simulink model "ELM_tictactoe_V2"  (R2021b)
settings: Solver=VariableStepAuto  StartTime=0.0  StopTime=inf  RelTol=1e-3
(part 1 of 136)
settings Model: Creator=benwa  LastModifiedBy=benwa
settings SolverCC: AutoInsertRateTranBlk=on

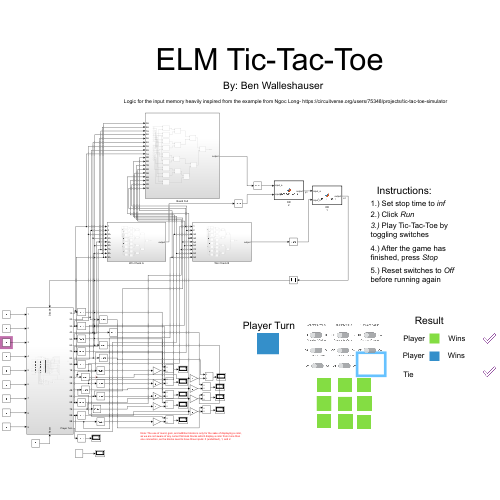
[thumbnail: Simulink's stored preview of the top-level diagram]
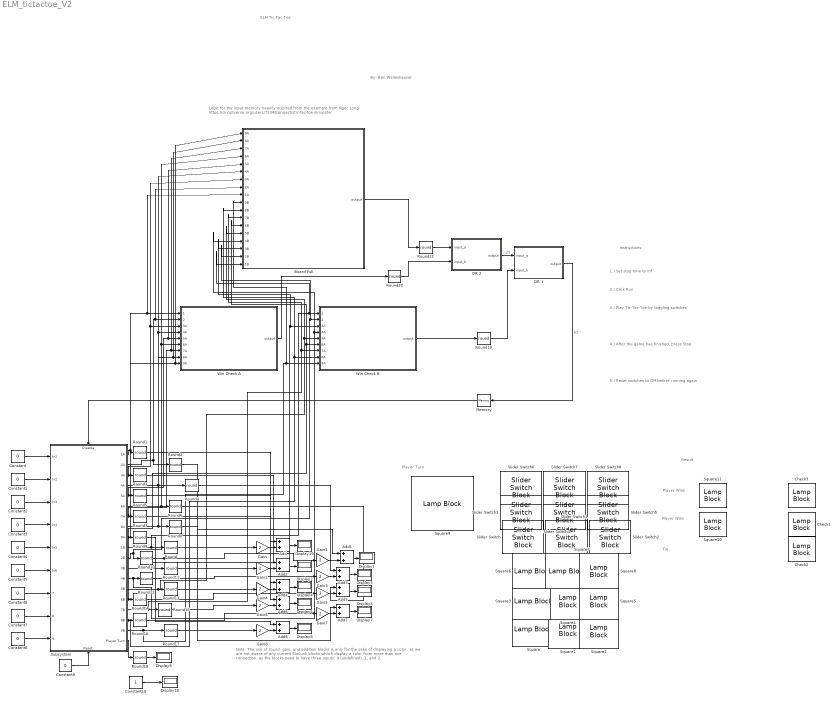
== system ELM_tictactoe_V2 ==
  note: Logic for the input memory heavily inspired from the example from Ngoc Long- https://circuitverse.org/users/75348/projects/tic-tac-toe-simulator
  note: By: Ben Walleshauser
  note: ELM Tic-Tac-Toe
  note: Note: The use of round, gain, and addition blocks is only for the sake of displaying a color, as we are not aware of any current Simlunk blocks whiich display a color from more than one connection, as the blocks need to have three inputs: 0 (undefined), 1, and 2.
  note: 1.) Set stop time to inf
  note: Instructions:
  note: Tie
  note: Player Wins
  note: Result
  note: Player Turn
  note: Player Wins
  note: 2.) Click Run
  note: 3.) Play Tic-Tac-Toe by toggling switches
  note: 4.) After the game has finished, press Stop
  note: 5.) Reset switches to Off before running again
  Add{,1..8} (9 alike) : Sum
  Board Full : Subsystem
  Check1 : LampBlock  LabelPosition=Hide  Icon=Check3
  Check2 : LampBlock  LabelPosition=Hide  Icon=Check3
  Check3 : LampBlock  LabelPosition=Hide  Icon=Check3
  Constant{,1..9} (10 alike) : Constant  Value=0
  Constant10 : Constant
  Display{1..10,19} (11 alike) : Display
  Gain{,1..8} (9 alike) : Gain  Gain=2
  Memory : Memory
  OR 1 : MATLAB Function  TreatAsAtomicUnit=on
  OR 2 : MATLAB Function  TreatAsAtomicUnit=on
  Round{,1..21} (22 alike) : Rounding  Operator=round
  Slider Switch{,1..8} (9 alike) : SliderSwitchBlock
      settings: Values={{'Off', 'On'}, [0 1]}
  Square{,1..11} (12 alike) : LampBlock  LabelPosition=Hide  Icon=Square
  Subsystem : Subsystem
      settings: PortSchema="{\"entries\":[{\"content\":{\"sides\":[{\"content\":{\"connectorIds\":[\"In1\",\"In2\",\"In3\",\"In4\",\"In5\",\"In6\",\"In7\",\"In8\",\"In9\"]},\"type\":\"ConnectorPlacement.EquallySpacedRectSide\",\"uuid\":\"24eea2ca-bc54-45b4-8ca7-8e6d0582f2d8\"},{\"content\":{\"connectorIds\":[\"Out1\",\"Out2\",\"Out3\",\"Out4\",\"Out5\",\"Out6\",\"Out7\",\"Out8\",\"Out9\",\"Out10\",\"Out11\",\"Out12\",\"Out13\",\"Out14\",\"Out15\",\"Out16\",\"Out17\",\"Out18\",\"Out19\"],\"side\":\"RIGHT\"},\"type\":\"ConnectorPlacement.EquallySpacedRectSide\",\"uuid\":\"dcdda681-f03f-4783-934e-bb305b550037\"},{\"content\":{\"connectorIds\":[\"In10\"],\"side\":\"TOP\"},\"type\":\"ConnectorPlacement.EquallySpacedRectSide\",\"uuid\":\"fbafddca-e088-423f-ae92-9e95b73c1056\"},{\"content\":{\"connectorIds\":[\"In11\"],\"side\":\"BOTTOM\"},\"type\":\"ConnectorPlacement.EquallySpacedRectSide\",\"uuid\":\"e1bf0a8c-befc-41e7-9839-13c2c519b1eb\"}]},\"type\":\"ConnectorPlacement.EquallySpacedConnector\",\"uuid\":\"afff88fe-c887-456a-b96a-e3a40750e04a\"}],\"packageUris\":[\"http://schema.mathworks.com/mf0/Connector/R2020b\"],\"version\":\"1.0\"}"
  Win Check A : Subsystem
  Win Check B : Subsystem
  wires:
  Constant/1 -> Subsystem/1(In1)
  Constant1/1 -> Subsystem/2(In2)
  Constant2/1 -> Subsystem/3(In3)
  Constant3/1 -> Subsystem/4(In4)
  Constant4/1 -> Subsystem/5(In5)
  Constant5/1 -> Subsystem/6(In6)
  Constant6/1 -> Subsystem/7(7)
  Constant7/1 -> Subsystem/8(8)
  Constant8/1 -> Subsystem/9(9)
  Constant9/1 -> Subsystem/11(Reset)
  Subsystem/1(1A) -> Round1/1, Board Full/9(1A), Win Check A/1(1)
  Subsystem/2(2A) -> Round2/1, Board Full/8(2A), Win Check A/2(2)
  Subsystem/3(3A) -> Board Full/7(3A), Win Check A/3(3A), Round3/1
  Subsystem/4(4A) -> Board Full/6(4A), Win Check A/4(4A), Round4/1
  Subsystem/5(5A) -> Board Full/5(5A), Win Check A/5(5A), Round5/1
  Subsystem/6(6A) -> Board Full/4(6A), Win Check A/6(6A), Round6/1
  Subsystem/7(7A) -> Board Full/3(7A), Win Check A/7(7A), Round7/1
  Subsystem/8(8A) -> Board Full/2(8A), Win Check A/8(8A), Round8/1
  Subsystem/9(9A) -> Round9/1, Board Full/1(9A), Win Check A/9(9A)
  Subsystem/10(1B) -> Win Check B/1(1), Board Full/18(1B), Round/1
  Subsystem/11(2B) -> Round10/1, Win Check B/2(2), Board Full/17(2B)
  Subsystem/12(3B) -> Win Check B/3(3A), Board Full/16(3B), Round11/1
  Subsystem/13(4B) -> Win Check B/4(4A), Board Full/15(4B), Round12/1
  Subsystem/14(5B) -> Win Check B/5(5A), Board Full/14(5B), Round13/1
  Subsystem/15(6B) -> Win Check B/6(6A), Board Full/13(6B), Round14/1
  Subsystem/16(7B) -> Win Check B/7(7A), Board Full/12(7B), Round15/1
  Round1/1 -> Add/1
  Round/1 -> Gain/1
  Gain/1 -> Add/2
  Add/1 -> Display19/1
  Gain1/1 -> Add1/2
  Gain2/1 -> Add2/2
  Gain3/1 -> Add3/2
  Gain4/1 -> Add4/2
  Gain5/1 -> Add5/2
  Gain6/1 -> Add6/2
  Gain7/1 -> Add7/2
  Gain8/1 -> Add8/2
  Round2/1 -> Add1/1
  Round5/1 -> Add4/1
  Round7/1 -> Add6/1
  Round9/1 -> Add8/1
  Round11/1 -> Gain2/1
  Round12/1 -> Gain3/1
  Round13/1 -> Gain4/1
  Round14/1 -> Gain5/1
  Round15/1 -> Gain6/1
  Round16/1 -> Gain7/1
  Round17/1 -> Gain8/1
  Round10/1 -> Gain1/1
  Round4/1 -> Add3/1
  Round3/1 -> Add2/1
  Round6/1 -> Add5/1
  Round8/1 -> Add7/1
  Add1/1 -> Display1/1
  Add2/1 -> Display2/1
  Add3/1 -> Display3/1
  Add4/1 -> Display4/1
  Add5/1 -> Display5/1
  Add6/1 -> Display6/1
  Add7/1 -> Display7/1
  Add8/1 -> Display8/1
  Subsystem/18(9B) -> Win Check B/9(9A), Board Full/10(9B), Round17/1
  Subsystem/17(8B) -> Round16/1, Win Check B/8(8A), Board Full/11(8B)
  OR 2/1(output) -> OR 1/1(input_a)  "p1"
  Board Full/1(output) -> Round21/1
  Win Check A/1(output) -> Round20/1
  Win Check B/1(output) -> Round19/1
  OR 1/1(output) -> Memory/1  "p1"
  Memory/1 -> Subsystem/10(Disable)
  Subsystem/19(Player Turn) -> Round18/1
  Round18/1 -> Display9/1
  Constant10/1 -> Display10/1
  Round19/1 -> OR 1/2(input_b)
  Round20/1 -> OR 2/2(input_b)
  Round21/1 -> OR 2/1(input_a)

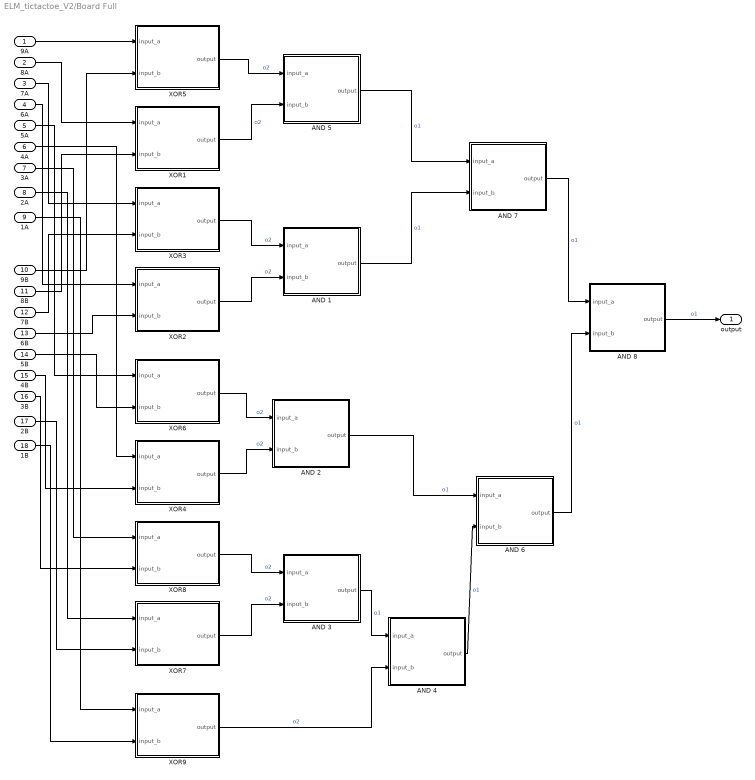
== system ELM_tictactoe_V2/Board Full ==
  9A : Inport
  8A : Inport  Port=2
  7A : Inport  Port=3
  6A : Inport  Port=4
  5A : Inport  Port=5
  4A : Inport  Port=6
  3A : Inport  Port=7
  2A : Inport  Port=8
  1A : Inport  Port=9
  9B : Inport  Port=10
  8B : Inport  Port=11
  7B : Inport  Port=12
  6B : Inport  Port=13
  5B : Inport  Port=14
  4B : Inport  Port=15
  3B : Inport  Port=16
  2B : Inport  Port=17
  1B : Inport  Port=18
  AND 1 : MATLAB Function  TreatAsAtomicUnit=on
  AND 2 : MATLAB Function  TreatAsAtomicUnit=on
  AND 3 : MATLAB Function  TreatAsAtomicUnit=on
  AND 4 : MATLAB Function  TreatAsAtomicUnit=on
  AND 5 : MATLAB Function  TreatAsAtomicUnit=on
  AND 6 : MATLAB Function  TreatAsAtomicUnit=on
  AND 7 : MATLAB Function  TreatAsAtomicUnit=on
  AND 8 : MATLAB Function  TreatAsAtomicUnit=on
  XOR1 : MATLAB Function  TreatAsAtomicUnit=on
  XOR2 : MATLAB Function  TreatAsAtomicUnit=on
  XOR3 : MATLAB Function  TreatAsAtomicUnit=on
  XOR4 : MATLAB Function  TreatAsAtomicUnit=on
  XOR5 : MATLAB Function  TreatAsAtomicUnit=on
  XOR6 : MATLAB Function  TreatAsAtomicUnit=on
  XOR7 : MATLAB Function  TreatAsAtomicUnit=on
  XOR8 : MATLAB Function  TreatAsAtomicUnit=on
  XOR9 : MATLAB Function  TreatAsAtomicUnit=on
  output : Outport
  wires:
  9A/1 -> XOR5/1(input_a)
  9B/1 -> XOR5/2(input_b)
  8A/1 -> XOR1/1(input_a)
  8B/1 -> XOR1/2(input_b)
  7A/1 -> XOR3/1(input_a)
  7B/1 -> XOR3/2(input_b)
  6A/1 -> XOR2/1(input_a)
  6B/1 -> XOR2/2(input_b)
  5A/1 -> XOR6/1(input_a)
  5B/1 -> XOR6/2(input_b)
  4A/1 -> XOR4/1(input_a)
  4B/1 -> XOR4/2(input_b)
  3A/1 -> XOR8/1(input_a)
  3B/1 -> XOR8/2(input_b)
  2A/1 -> XOR7/1(input_a)
  2B/1 -> XOR7/2(input_b)
  1A/1 -> XOR9/1(input_a)
  1B/1 -> XOR9/2(input_b)
  XOR5/1(output) -> AND 5/1(input_a)  "o2"
  XOR1/1(output) -> AND 5/2(input_b)  "o2"
  XOR3/1(output) -> AND 1/1(input_a)  "o2"
  XOR2/1(output) -> AND 1/2(input_b)  "o2"
  XOR6/1(output) -> AND 2/1(input_a)  "o2"
  XOR4/1(output) -> AND 2/2(input_b)  "o2"
  XOR8/1(output) -> AND 3/1(input_a)  "o2"
  XOR7/1(output) -> AND 3/2(input_b)  "o2"
  XOR9/1(output) -> AND 4/2(input_b)  "o2"
  AND 3/1(output) -> AND 4/1(input_a)  "o1"
  AND 1/1(output) -> AND 7/2(input_b)  "o1"
  AND 5/1(output) -> AND 7/1(input_a)  "o1"
  AND 2/1(output) -> AND 6/1(input_a)  "o1"
  AND 4/1(output) -> AND 6/2(input_b)  "o1"
  AND 6/1(output) -> AND 8/2(input_b)  "o1"
  AND 7/1(output) -> AND 8/1(input_a)  "o1"
  AND 8/1(output) -> output/1  "o1"

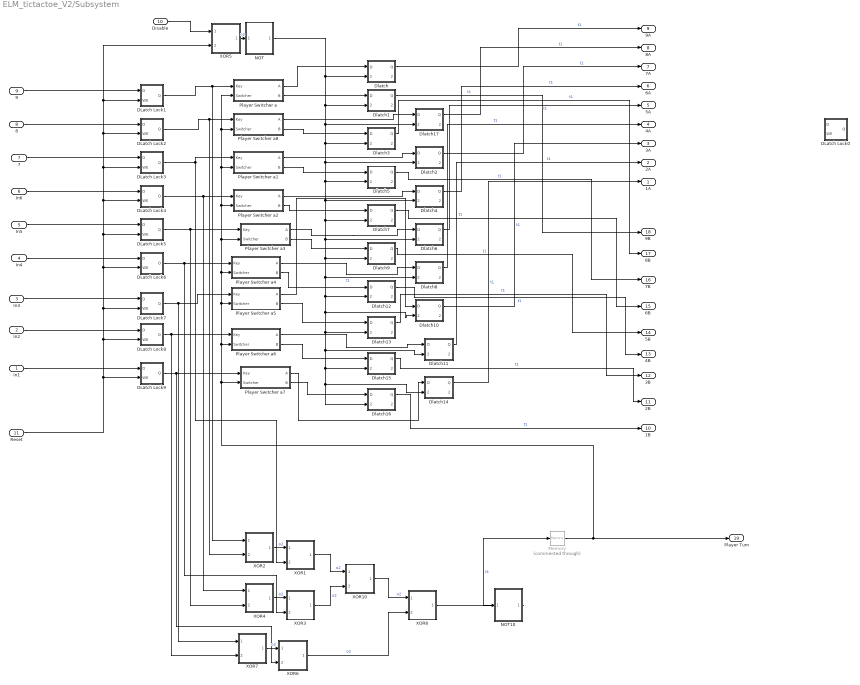
== system ELM_tictactoe_V2/Subsystem ==
  In1 : Inport
  In2 : Inport  Port=2
  In3 : Inport  Port=3
  In4 : Inport  Port=4
  In5 : Inport  Port=5
  In6 : Inport  Port=6
  7 : Inport  Port=7
  8 : Inport  Port=8
  9 : Inport  Port=9
  Disable : Inport  Port=10
  Reset : Inport  Port=11
  DLatch Lock0 : Subsystem
  DLatch Lock1 : Subsystem
  DLatch Lock2 : Subsystem
  DLatch Lock3 : Subsystem
  DLatch Lock4 : Subsystem
  DLatch Lock5 : Subsystem
  DLatch Lock6 : Subsystem
  DLatch Lock7 : Subsystem
  DLatch Lock8 : Subsystem
  DLatch Lock9 : Subsystem
  Dlatch : Subsystem
  Dlatch1 : Subsystem
  Dlatch10 : Subsystem
  Dlatch11 : Subsystem
  Dlatch12 : Subsystem
  Dlatch13 : Subsystem
  Dlatch14 : Subsystem
  Dlatch15 : Subsystem
  Dlatch16 : Subsystem
  Dlatch17 : Subsystem
  Dlatch2 : Subsystem
  Dlatch3 : Subsystem
  Dlatch4 : Subsystem
  Dlatch5 : Subsystem
  Dlatch6 : Subsystem
  Dlatch7 : Subsystem
  Dlatch8 : Subsystem
  Dlatch9 : Subsystem
  Memory : Memory  Commented=through
  NOT : MATLAB Function  TreatAsAtomicUnit=on
  NOT10 : MATLAB Function  TreatAsAtomicUnit=on
  Player Switcher a : Subsystem
  Player Switcher a1 : Subsystem
  Player Switcher a2 : Subsystem
  Player Switcher a3 : Subsystem
  Player Switcher a4 : Subsystem
  Player Switcher a5 : Subsystem
  Player Switcher a6 : Subsystem
  Player Switcher a7 : Subsystem
  Player Switcher a8 : Subsystem
  XOR1 : MATLAB Function  TreatAsAtomicUnit=on
  XOR10 : MATLAB Function  TreatAsAtomicUnit=on
  XOR2 : MATLAB Function  TreatAsAtomicUnit=on
  XOR3 : MATLAB Function  TreatAsAtomicUnit=on
  XOR4 : MATLAB Function  TreatAsAtomicUnit=on
  XOR5 : MATLAB Function  TreatAsAtomicUnit=on
  XOR6 : MATLAB Function  TreatAsAtomicUnit=on
  XOR7 : MATLAB Function  TreatAsAtomicUnit=on
  XOR8 : MATLAB Function  TreatAsAtomicUnit=on
  1A : Outport
  2A : Outport  Port=2
  3A : Outport  Port=3
  4A : Outport  Port=4
  5A : Outport  Port=5
  6A : Outport  Port=6
  7A : Outport  Port=7
  8A : Outport  Port=8
  9A : Outport  Port=9
  1B : Outport  Port=10
  2B : Outport  Port=11
  3B : Outport  Port=12
  4B : Outport  Port=13
  5B : Outport  Port=14
  6B : Outport  Port=15
  7B : Outport  Port=16
  8B : Outport  Port=17
  9B : Outport  Port=18
  Player Turn : Outport  Port=19
  wires:
  XOR5/1(output) -> NOT/1(input_a)  "o2"
  Disable/1 -> XOR5/1(input_a)
  Reset/1 -> DLatch Lock9/2(WE), DLatch Lock8/2(WE), DLatch Lock7/2(WE), DLatch Lock6/2(WE), DLatch Lock5/2(WE), DLatch Lock4/2(WE), DLatch Lock3/2(WE), DLatch Lock2/2(WE), XOR5/2(input_b), DLatch Lock1/2(WE)
  9/1 -> DLatch Lock1/1(D)
  8/1 -> DLatch Lock2/1(D)
  7/1 -> DLatch Lock3/1(D)
  In6/1 -> DLatch Lock4/1(D)
  In5/1 -> DLatch Lock5/1(D)
  In4/1 -> DLatch Lock6/1(D)
  In3/1 -> DLatch Lock7/1(D)
  In2/1 -> DLatch Lock8/1(D)
  In1/1 -> DLatch Lock9/1(D)
  DLatch Lock1/1(Q) -> Player Switcher a/1(Key), XOR2/1(input_a)
  DLatch Lock2/1(Q) -> Player Switcher a8/1(Key), XOR2/2(input_b)
  DLatch Lock3/1(Q) -> Player Switcher a1/1(Key), XOR1/2(input_b)
  DLatch Lock5/1(Q) -> Player Switcher a3/1(Key), XOR4/2(input_b)
  DLatch Lock7/1(Q) -> Player Switcher a5/1(Key), XOR7/1(input_a)
  DLatch Lock8/1(Q) -> Player Switcher a6/1(Key), XOR7/2(input_b)
  DLatch Lock9/1(Q) -> Player Switcher a7/1(Key), XOR6/2(input_b)
  NOT/1(output) -> Dlatch/2(Clock), Dlatch1/2(Clock), Dlatch17/2(Clock), Dlatch3/2(Clock), Dlatch2/2(Clock), Dlatch5/2(Clock), Dlatch4/2(Clock), Dlatch7/2(Clock), Dlatch6/2(Clock), Dlatch9/2(Clock), Dlatch8/2(Clock), Dlatch12/2(Clock), Dlatch10/2(Clock), Dlatch13/2(Clock), Dlatch11/2(Clock), Dlatch15/2(Clock), Dlatch16/2(Clock), Dlatch14/2(Clock)  "t1"
  Player Switcher a/1(A) -> Dlatch/1(D)
  Player Switcher a/2(B) -> Dlatch1/1(D)
  Dlatch/1(Q) -> 9A/1  "t1"
  Dlatch1/1(Q) -> 9B/1  "t1"
  Player Switcher a8/1(A) -> Dlatch17/1(D)
  Player Switcher a8/2(B) -> Dlatch3/1(D)
  Dlatch17/1(Q) -> 8A/1  "t1"
  Dlatch3/1(Q) -> 8B/1  "t1"
  Player Switcher a1/1(A) -> Dlatch2/1(D)
  Dlatch2/1(Q) -> 7A/1  "t1"
  Player Switcher a1/2(B) -> Dlatch5/1(D)
  Dlatch5/1(Q) -> 7B/1  "t1"
  Player Switcher a2/1(A) -> Dlatch4/1(D)
  Player Switcher a2/2(B) -> Dlatch7/1(D)
  Dlatch4/1(Q) -> 6A/1  "t1"
  Dlatch7/1(Q) -> 6B/1  "t1"
  Player Switcher a3/1(A) -> Dlatch6/1(D)
  Player Switcher a3/2(B) -> Dlatch9/1(D)
  Dlatch6/1(Q) -> 5A/1  "t1"
  Dlatch9/1(Q) -> 5B/1  "t1"
  Player Switcher a4/1(A) -> Dlatch8/1(D)
  Player Switcher a4/2(B) -> Dlatch12/1(D)
  Dlatch8/1(Q) -> 4A/1  "t1"
  Player Switcher a5/1(A) -> Dlatch10/1(D)
  Player Switcher a5/2(B) -> Dlatch13/1(D)
  Dlatch10/1(Q) -> 3A/1  "t1"
  Dlatch13/1(Q) -> 3B/1  "t1"
  Player Switcher a6/1(A) -> Dlatch11/1(D)
  Player Switcher a6/2(B) -> Dlatch15/1(D)
  Dlatch11/1(Q) -> 2A/1  "t1"
  Dlatch15/1(Q) -> 2B/1  "t1"
  Player Switcher a7/1(A) -> Dlatch14/1(D)
  Player Switcher a7/2(B) -> Dlatch16/1(D)
  Dlatch14/1(Q) -> 1A/1  "t1"
  Dlatch16/1(Q) -> 1B/1  "t1"
  Dlatch12/1(Q) -> 4B/1  "t1"
  Memory/1 -> Player Turn/1, Player Switcher a7/2(Switcher), Player Switcher a6/2(Switcher), Player Switcher a5/2(Switcher), Player Switcher a4/2(Switcher), Player Switcher a3/2(Switcher), Player Switcher a2/2(Switcher), Player Switcher a1/2(Switcher), Player Switcher a8/2(Switcher), Player Switcher a/2(Switcher)
  XOR10/1(output) -> XOR8/1(input_a)  "o2"
  XOR1/1(output) -> XOR10/1(input_a)  "o2"
  XOR2/1(output) -> XOR1/1(input_a)  "o2"
  XOR3/1(output) -> XOR10/2(input_b)  "o2"
  XOR7/1(output) -> XOR6/1(input_a)  "o2"
  XOR4/1(output) -> XOR3/1(input_a)  "o2"
  XOR6/1(output) -> XOR8/2(input_b)  "o2"
  DLatch Lock4/1(Q) -> Player Switcher a2/1(Key), XOR4/1(input_a)
  XOR8/1(output) -> NOT10/1(input_a)
  DLatch Lock6/1(Q) -> Player Switcher a4/1(Key), XOR3/2(input_b)
  NOT10/1(output) -> Memory/1  "t1"

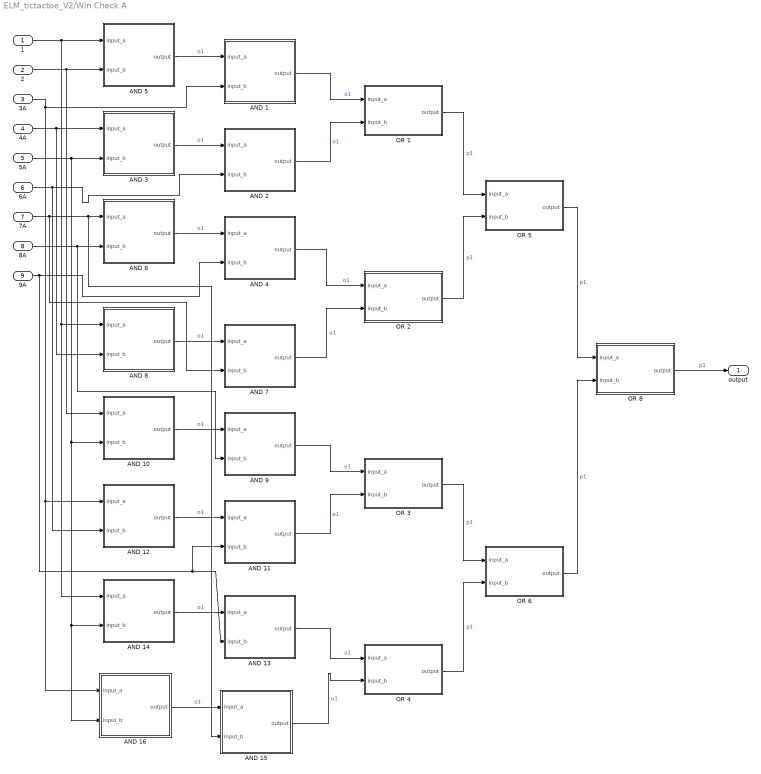
== system ELM_tictactoe_V2/Win Check A ==
  1 : Inport
  2 : Inport  Port=2
  3A : Inport  Port=3
  4A : Inport  Port=4
  5A : Inport  Port=5
  6A : Inport  Port=6
  7A : Inport  Port=7
  8A : Inport  Port=8
  9A : Inport  Port=9
  AND 1 : MATLAB Function  TreatAsAtomicUnit=on
  AND 10 : MATLAB Function  TreatAsAtomicUnit=on
  AND 11 : MATLAB Function  TreatAsAtomicUnit=on
  AND 12 : MATLAB Function  TreatAsAtomicUnit=on
  AND 13 : MATLAB Function  TreatAsAtomicUnit=on
  AND 14 : MATLAB Function  TreatAsAtomicUnit=on
  AND 15 : MATLAB Function  TreatAsAtomicUnit=on
  AND 16 : MATLAB Function  TreatAsAtomicUnit=on
  AND 2 : MATLAB Function  TreatAsAtomicUnit=on
  AND 3 : MATLAB Function  TreatAsAtomicUnit=on
  AND 4 : MATLAB Function  TreatAsAtomicUnit=on
  AND 5 : MATLAB Function  TreatAsAtomicUnit=on
  AND 6 : MATLAB Function  TreatAsAtomicUnit=on
  AND 7 : MATLAB Function  TreatAsAtomicUnit=on
  AND 8 : MATLAB Function  TreatAsAtomicUnit=on
  AND 9 : MATLAB Function  TreatAsAtomicUnit=on
  OR 1 : MATLAB Function  TreatAsAtomicUnit=on
  OR 2 : MATLAB Function  TreatAsAtomicUnit=on
  OR 3 : MATLAB Function  TreatAsAtomicUnit=on
  OR 4 : MATLAB Function  TreatAsAtomicUnit=on
  OR 5 : MATLAB Function  TreatAsAtomicUnit=on
  OR 6 : MATLAB Function  TreatAsAtomicUnit=on
  OR 8 : MATLAB Function  TreatAsAtomicUnit=on
  output : Outport
  wires:
  2/1 -> AND 10/1(input_a), AND 5/2(input_b)
  AND 5/1(output) -> AND 1/1(input_a)  "o1"
  3A/1 -> AND 1/2(input_b), AND 16/1(input_a), AND 12/1(input_a)
  AND 3/1(output) -> AND 2/1(input_a)  "o1"
  6A/1 -> AND 12/2(input_b), AND 2/2(input_b)
  5A/1 -> AND 3/2(input_b), AND 10/2(input_b), AND 16/2(input_b), AND 14/2(input_b)
  AND 6/1(output) -> AND 4/1(input_a)  "o1"
  9A/1 -> AND 4/2(input_b), AND 13/2(input_b), AND 11/2(input_b)
  8A/1 -> AND 9/2(input_b), AND 6/2(input_b)
  AND 8/1(output) -> AND 7/1(input_a)  "o1"
  1/1 -> AND 14/1(input_a), AND 8/1(input_a), AND 5/1(input_a)
  7A/1 -> AND 7/2(input_b), AND 15/2(input_b), AND 6/1(input_a)
  4A/1 -> AND 8/2(input_b), AND 3/1(input_a)
  AND 10/1(output) -> AND 9/1(input_a)  "o1"
  AND 12/1(output) -> AND 11/1(input_a)  "o1"
  AND 14/1(output) -> AND 13/1(input_a)  "o1"
  AND 16/1(output) -> AND 15/1(input_a)  "o1"
  AND 15/1(output) -> OR 4/2(input_b)  "o1"
  AND 13/1(output) -> OR 4/1(input_a)  "o1"
  AND 11/1(output) -> OR 3/2(input_b)  "o1"
  AND 9/1(output) -> OR 3/1(input_a)  "o1"
  AND 7/1(output) -> OR 2/2(input_b)  "o1"
  AND 4/1(output) -> OR 2/1(input_a)  "o1"
  AND 2/1(output) -> OR 1/2(input_b)  "o1"
  AND 1/1(output) -> OR 1/1(input_a)  "o1"
  OR 4/1(output) -> OR 6/2(input_b)  "p1"
  OR 3/1(output) -> OR 6/1(input_a)  "p1"
  OR 1/1(output) -> OR 5/1(input_a)  "p1"
  OR 6/1(output) -> OR 8/2(input_b)  "p1"
  OR 5/1(output) -> OR 8/1(input_a)  "p1"
  OR 8/1(output) -> output/1  "p1"
  OR 2/1(output) -> OR 5/2(input_b)  "p1"

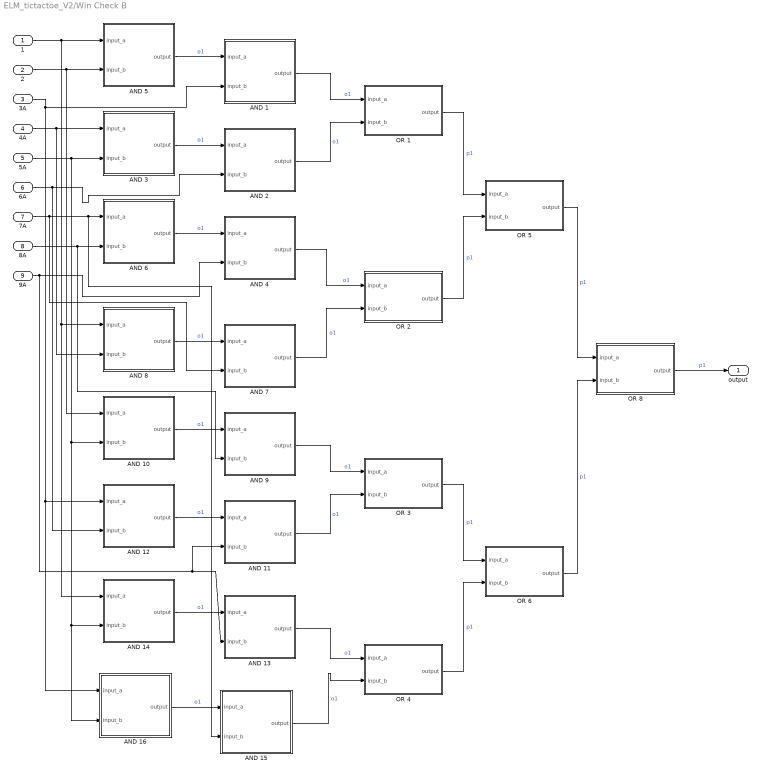
== system ELM_tictactoe_V2/Win Check B ==
  1 : Inport
  2 : Inport  Port=2
  3A : Inport  Port=3
  4A : Inport  Port=4
  5A : Inport  Port=5
  6A : Inport  Port=6
  7A : Inport  Port=7
  8A : Inport  Port=8
  9A : Inport  Port=9
  AND 1 : MATLAB Function  TreatAsAtomicUnit=on
  AND 10 : MATLAB Function  TreatAsAtomicUnit=on
  AND 11 : MATLAB Function  TreatAsAtomicUnit=on
  AND 12 : MATLAB Function  TreatAsAtomicUnit=on
  AND 13 : MATLAB Function  TreatAsAtomicUnit=on
  AND 14 : MATLAB Function  TreatAsAtomicUnit=on
  AND 15 : MATLAB Function  TreatAsAtomicUnit=on
  AND 16 : MATLAB Function  TreatAsAtomicUnit=on
  AND 2 : MATLAB Function  TreatAsAtomicUnit=on
  AND 3 : MATLAB Function  TreatAsAtomicUnit=on
  AND 4 : MATLAB Function  TreatAsAtomicUnit=on
  AND 5 : MATLAB Function  TreatAsAtomicUnit=on
  AND 6 : MATLAB Function  TreatAsAtomicUnit=on
  AND 7 : MATLAB Function  TreatAsAtomicUnit=on
  AND 8 : MATLAB Function  TreatAsAtomicUnit=on
  AND 9 : MATLAB Function  TreatAsAtomicUnit=on
  OR 1 : MATLAB Function  TreatAsAtomicUnit=on
  OR 2 : MATLAB Function  TreatAsAtomicUnit=on
  OR 3 : MATLAB Function  TreatAsAtomicUnit=on
  OR 4 : MATLAB Function  TreatAsAtomicUnit=on
  OR 5 : MATLAB Function  TreatAsAtomicUnit=on
  OR 6 : MATLAB Function  TreatAsAtomicUnit=on
  OR 8 : MATLAB Function  TreatAsAtomicUnit=on
  output : Outport
  wires:
  2/1 -> AND 10/1(input_a), AND 5/2(input_b)
  AND 5/1(output) -> AND 1/1(input_a)  "o1"
  3A/1 -> AND 1/2(input_b), AND 16/1(input_a), AND 12/1(input_a)
  AND 3/1(output) -> AND 2/1(input_a)  "o1"
  6A/1 -> AND 12/2(input_b), AND 2/2(input_b)
  5A/1 -> AND 3/2(input_b), AND 10/2(input_b), AND 16/2(input_b), AND 14/2(input_b)
  AND 6/1(output) -> AND 4/1(input_a)  "o1"
  9A/1 -> AND 4/2(input_b), AND 13/2(input_b), AND 11/2(input_b)
  8A/1 -> AND 9/2(input_b), AND 6/2(input_b)
  AND 8/1(output) -> AND 7/1(input_a)  "o1"
  1/1 -> AND 14/1(input_a), AND 8/1(input_a), AND 5/1(input_a)
  7A/1 -> AND 7/2(input_b), AND 15/2(input_b), AND 6/1(input_a)
  4A/1 -> AND 8/2(input_b), AND 3/1(input_a)
  AND 10/1(output) -> AND 9/1(input_a)  "o1"
  AND 12/1(output) -> AND 11/1(input_a)  "o1"
  AND 14/1(output) -> AND 13/1(input_a)  "o1"
  AND 16/1(output) -> AND 15/1(input_a)  "o1"
  AND 15/1(output) -> OR 4/2(input_b)  "o1"
  AND 13/1(output) -> OR 4/1(input_a)  "o1"
  AND 11/1(output) -> OR 3/2(input_b)  "o1"
  AND 9/1(output) -> OR 3/1(input_a)  "o1"
  AND 7/1(output) -> OR 2/2(input_b)  "o1"
  AND 4/1(output) -> OR 2/1(input_a)  "o1"
  AND 2/1(output) -> OR 1/2(input_b)  "o1"
  AND 1/1(output) -> OR 1/1(input_a)  "o1"
  OR 4/1(output) -> OR 6/2(input_b)  "p1"
  OR 3/1(output) -> OR 6/1(input_a)  "p1"
  OR 1/1(output) -> OR 5/1(input_a)  "p1"
  OR 6/1(output) -> OR 8/2(input_b)  "p1"
  OR 5/1(output) -> OR 8/1(input_a)  "p1"
  OR 8/1(output) -> output/1  "p1"
  OR 2/1(output) -> OR 5/2(input_b)  "p1"

== system ELM_tictactoe_V2/Subsystem/DLatch Lock0 ==
  D : Inport
  WE : Inport  Port=2
  Dlatch : Subsystem
  NOT : MATLAB Function  TreatAsAtomicUnit=on
  OR 2 : MATLAB Function  TreatAsAtomicUnit=on
  Q : Outport
  wires:
  Dlatch/1(Q) -> NOT/1(input_a)
  NOT/1(output) -> Q/1  "t1"
  D/1 -> Dlatch/2(D), OR 2/1(input_a)
  WE/1 -> OR 2/2(input_b)
  OR 2/1(output) -> Dlatch/1(Clock)  "p1"

== system ELM_tictactoe_V2/Subsystem/DLatch Lock1 ==
  D : Inport
  WE : Inport  Port=2
  Dlatch : Subsystem
  OR 2 : MATLAB Function  TreatAsAtomicUnit=on
  Q : Outport
  wires:
  Dlatch/1(Q) -> Q/1  "t1"
  D/1 -> Dlatch/1(D), OR 2/1(input_a)
  WE/1 -> OR 2/2(input_b)
  OR 2/1(output) -> Dlatch/2(Clock)  "p1"

== system ELM_tictactoe_V2/Subsystem/DLatch Lock2 ==
  D : Inport
  WE : Inport  Port=2
  Dlatch : Subsystem
  OR 2 : MATLAB Function  TreatAsAtomicUnit=on
  Q : Outport
  wires:
  Dlatch/1(Q) -> Q/1  "t1"
  D/1 -> Dlatch/1(D), OR 2/1(input_a)
  WE/1 -> OR 2/2(input_b)
  OR 2/1(output) -> Dlatch/2(Clock)  "p1"

== system ELM_tictactoe_V2/Subsystem/DLatch Lock3 ==
  D : Inport
  WE : Inport  Port=2
  Dlatch : Subsystem
  OR 2 : MATLAB Function  TreatAsAtomicUnit=on
  Q : Outport
  wires:
  Dlatch/1(Q) -> Q/1  "t1"
  D/1 -> Dlatch/1(D), OR 2/1(input_a)
  WE/1 -> OR 2/2(input_b)
  OR 2/1(output) -> Dlatch/2(Clock)  "p1"

== system ELM_tictactoe_V2/Subsystem/DLatch Lock4 ==
  D : Inport
  WE : Inport  Port=2
  Dlatch : Subsystem
  OR 2 : MATLAB Function  TreatAsAtomicUnit=on
  Q : Outport
  wires:
  Dlatch/1(Q) -> Q/1  "t1"
  D/1 -> Dlatch/1(D), OR 2/1(input_a)
  WE/1 -> OR 2/2(input_b)
  OR 2/1(output) -> Dlatch/2(Clock)  "p1"

== system ELM_tictactoe_V2/Subsystem/DLatch Lock5 ==
  D : Inport
  WE : Inport  Port=2
  Dlatch : Subsystem
  OR 2 : MATLAB Function  TreatAsAtomicUnit=on
  Q : Outport
  wires:
  Dlatch/1(Q) -> Q/1  "t1"
  D/1 -> Dlatch/1(D), OR 2/1(input_a)
  WE/1 -> OR 2/2(input_b)
  OR 2/1(output) -> Dlatch/2(Clock)  "p1"

== system ELM_tictactoe_V2/Subsystem/DLatch Lock6 ==
  D : Inport
  WE : Inport  Port=2
  Dlatch : Subsystem
  OR 2 : MATLAB Function  TreatAsAtomicUnit=on
  Q : Outport
  wires:
  Dlatch/1(Q) -> Q/1  "t1"
  D/1 -> Dlatch/1(D), OR 2/1(input_a)
  WE/1 -> OR 2/2(input_b)
  OR 2/1(output) -> Dlatch/2(Clock)  "p1"

== system ELM_tictactoe_V2/Subsystem/DLatch Lock7 ==
  D : Inport
  WE : Inport  Port=2
  Dlatch : Subsystem
  OR 2 : MATLAB Function  TreatAsAtomicUnit=on
  Q : Outport
  wires:
  Dlatch/1(Q) -> Q/1  "t1"
  D/1 -> Dlatch/1(D), OR 2/1(input_a)
  WE/1 -> OR 2/2(input_b)
  OR 2/1(output) -> Dlatch/2(Clock)  "p1"

== system ELM_tictactoe_V2/Subsystem/DLatch Lock8 ==
  D : Inport
  WE : Inport  Port=2
  Dlatch : Subsystem
  OR 2 : MATLAB Function  TreatAsAtomicUnit=on
  Q : Outport
  wires:
  Dlatch/1(Q) -> Q/1  "t1"
  D/1 -> Dlatch/1(D), OR 2/1(input_a)
  WE/1 -> OR 2/2(input_b)
  OR 2/1(output) -> Dlatch/2(Clock)  "p1"

== system ELM_tictactoe_V2/Subsystem/DLatch Lock9 ==
  D : Inport
  WE : Inport  Port=2
  Dlatch : Subsystem
  OR 2 : MATLAB Function  TreatAsAtomicUnit=on
  Q : Outport
  wires:
  Dlatch/1(Q) -> Q/1  "t1"
  D/1 -> Dlatch/1(D), OR 2/1(input_a)
  WE/1 -> OR 2/2(input_b)
  OR 2/1(output) -> Dlatch/2(Clock)  "p1"

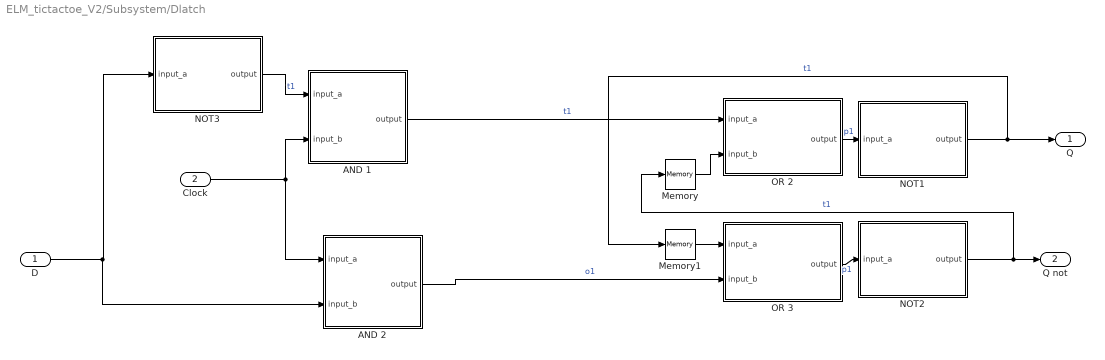
== system ELM_tictactoe_V2/Subsystem/Dlatch ==
  D : Inport
  Clock : Inport  Port=2
  AND 1 : MATLAB Function  TreatAsAtomicUnit=on
  AND 2 : MATLAB Function  TreatAsAtomicUnit=on
  Memory : Memory  InitialCondition=1  LinearizeAsDelay=on
  Memory1 : Memory  LinearizeAsDelay=on
  NOT1 : MATLAB Function  TreatAsAtomicUnit=on
  NOT2 : MATLAB Function  TreatAsAtomicUnit=on
  NOT3 : MATLAB Function  TreatAsAtomicUnit=on
  OR 2 : MATLAB Function  TreatAsAtomicUnit=on
  OR 3 : MATLAB Function  TreatAsAtomicUnit=on
  Q : Outport
  Q not : Outport  Port=2
  wires:
  D/1 -> NOT3/1(input_a), AND 2/2(input_b)
  NOT3/1(output) -> AND 1/1(input_a)  "t1"
  Clock/1 -> AND 1/2(input_b), AND 2/1(input_a)
  OR 2/1(output) -> NOT1/1(input_a)  "p1"
  OR 3/1(output) -> NOT2/1(input_a)  "p1"
  AND 2/1(output) -> OR 3/2(input_b)  "o1"
  NOT1/1(output) -> Memory1/1, Q/1  "t1"
  NOT2/1(output) -> Memory/1, Q not/1  "t1"
  AND 1/1(output) -> OR 2/1(input_a)  "t1"
  Memory/1 -> OR 2/2(input_b)
  Memory1/1 -> OR 3/1(input_a)

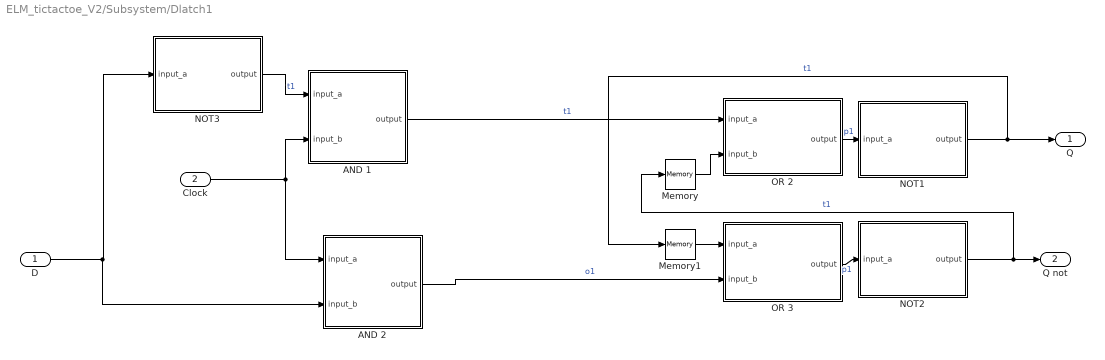
== system ELM_tictactoe_V2/Subsystem/Dlatch1 ==
  D : Inport
  Clock : Inport  Port=2
  AND 1 : MATLAB Function  TreatAsAtomicUnit=on
  AND 2 : MATLAB Function  TreatAsAtomicUnit=on
  Memory : Memory  InitialCondition=1  LinearizeAsDelay=on
  Memory1 : Memory  LinearizeAsDelay=on
  NOT1 : MATLAB Function  TreatAsAtomicUnit=on
  NOT2 : MATLAB Function  TreatAsAtomicUnit=on
  NOT3 : MATLAB Function  TreatAsAtomicUnit=on
  OR 2 : MATLAB Function  TreatAsAtomicUnit=on
  OR 3 : MATLAB Function  TreatAsAtomicUnit=on
  Q : Outport
  Q not : Outport  Port=2
  wires:
  D/1 -> NOT3/1(input_a), AND 2/2(input_b)
  NOT3/1(output) -> AND 1/1(input_a)  "t1"
  Clock/1 -> AND 1/2(input_b), AND 2/1(input_a)
  OR 2/1(output) -> NOT1/1(input_a)  "p1"
  OR 3/1(output) -> NOT2/1(input_a)  "p1"
  AND 2/1(output) -> OR 3/2(input_b)  "o1"
  NOT1/1(output) -> Memory1/1, Q/1  "t1"
  NOT2/1(output) -> Memory/1, Q not/1  "t1"
  AND 1/1(output) -> OR 2/1(input_a)  "t1"
  Memory/1 -> OR 2/2(input_b)
  Memory1/1 -> OR 3/1(input_a)

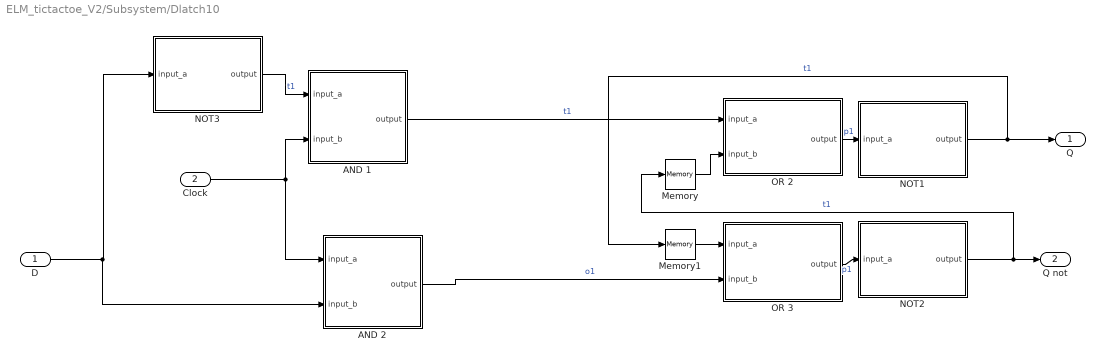
== system ELM_tictactoe_V2/Subsystem/Dlatch10 ==
  D : Inport
  Clock : Inport  Port=2
  AND 1 : MATLAB Function  TreatAsAtomicUnit=on
  AND 2 : MATLAB Function  TreatAsAtomicUnit=on
  Memory : Memory  InitialCondition=1  LinearizeAsDelay=on
  Memory1 : Memory  LinearizeAsDelay=on
  NOT1 : MATLAB Function  TreatAsAtomicUnit=on
  NOT2 : MATLAB Function  TreatAsAtomicUnit=on
  NOT3 : MATLAB Function  TreatAsAtomicUnit=on
  OR 2 : MATLAB Function  TreatAsAtomicUnit=on
  OR 3 : MATLAB Function  TreatAsAtomicUnit=on
  Q : Outport
  Q not : Outport  Port=2
  wires:
  D/1 -> NOT3/1(input_a), AND 2/2(input_b)
  NOT3/1(output) -> AND 1/1(input_a)  "t1"
  Clock/1 -> AND 1/2(input_b), AND 2/1(input_a)
  OR 2/1(output) -> NOT1/1(input_a)  "p1"
  OR 3/1(output) -> NOT2/1(input_a)  "p1"
  AND 2/1(output) -> OR 3/2(input_b)  "o1"
  NOT1/1(output) -> Memory1/1, Q/1  "t1"
  NOT2/1(output) -> Memory/1, Q not/1  "t1"
  AND 1/1(output) -> OR 2/1(input_a)  "t1"
  Memory/1 -> OR 2/2(input_b)
  Memory1/1 -> OR 3/1(input_a)

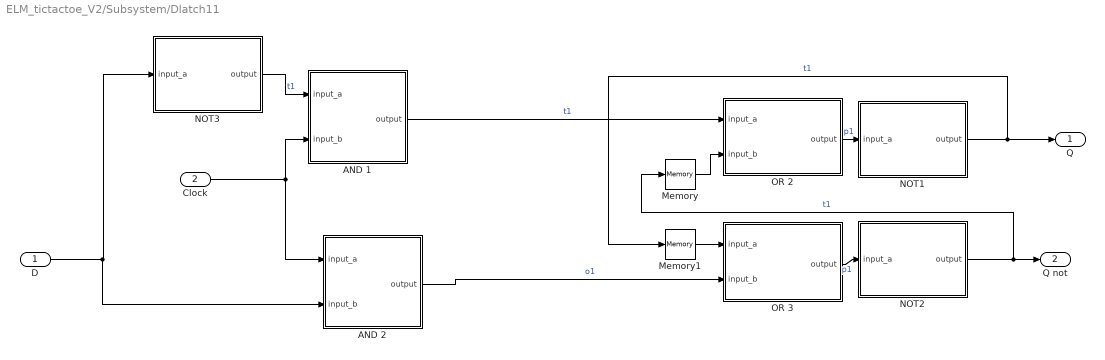
== system ELM_tictactoe_V2/Subsystem/Dlatch11 ==
  D : Inport
  Clock : Inport  Port=2
  AND 1 : MATLAB Function  TreatAsAtomicUnit=on
  AND 2 : MATLAB Function  TreatAsAtomicUnit=on
  Memory : Memory  InitialCondition=1  LinearizeAsDelay=on
  Memory1 : Memory  LinearizeAsDelay=on
  NOT1 : MATLAB Function  TreatAsAtomicUnit=on
  NOT2 : MATLAB Function  TreatAsAtomicUnit=on
  NOT3 : MATLAB Function  TreatAsAtomicUnit=on
  OR 2 : MATLAB Function  TreatAsAtomicUnit=on
  OR 3 : MATLAB Function  TreatAsAtomicUnit=on
  Q : Outport
  Q not : Outport  Port=2
  wires:
  D/1 -> NOT3/1(input_a), AND 2/2(input_b)
  NOT3/1(output) -> AND 1/1(input_a)  "t1"
  Clock/1 -> AND 1/2(input_b), AND 2/1(input_a)
  OR 2/1(output) -> NOT1/1(input_a)  "p1"
  OR 3/1(output) -> NOT2/1(input_a)  "p1"
  AND 2/1(output) -> OR 3/2(input_b)  "o1"
  NOT1/1(output) -> Memory1/1, Q/1  "t1"
  NOT2/1(output) -> Memory/1, Q not/1  "t1"
  AND 1/1(output) -> OR 2/1(input_a)  "t1"
  Memory/1 -> OR 2/2(input_b)
  Memory1/1 -> OR 3/1(input_a)

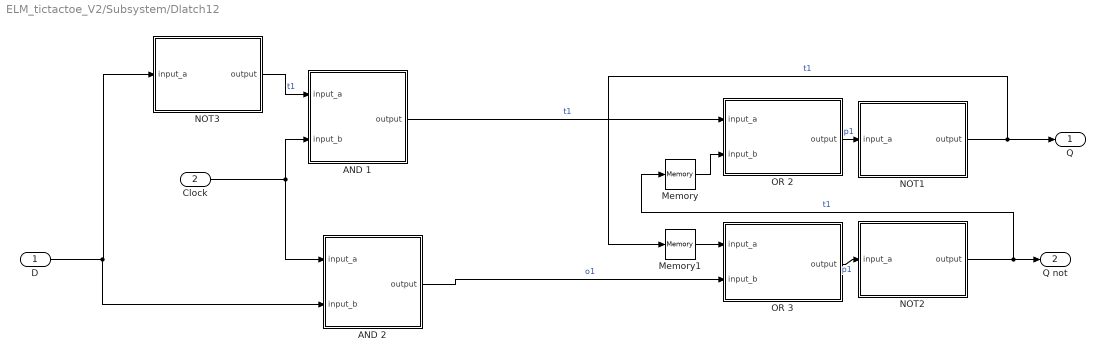
== system ELM_tictactoe_V2/Subsystem/Dlatch12 ==
  D : Inport
  Clock : Inport  Port=2
  AND 1 : MATLAB Function  TreatAsAtomicUnit=on
  AND 2 : MATLAB Function  TreatAsAtomicUnit=on
  Memory : Memory  InitialCondition=1  LinearizeAsDelay=on
  Memory1 : Memory  LinearizeAsDelay=on
  NOT1 : MATLAB Function  TreatAsAtomicUnit=on
  NOT2 : MATLAB Function  TreatAsAtomicUnit=on
  NOT3 : MATLAB Function  TreatAsAtomicUnit=on
  OR 2 : MATLAB Function  TreatAsAtomicUnit=on
  OR 3 : MATLAB Function  TreatAsAtomicUnit=on
  Q : Outport
  Q not : Outport  Port=2
  wires:
  D/1 -> NOT3/1(input_a), AND 2/2(input_b)
  NOT3/1(output) -> AND 1/1(input_a)  "t1"
  Clock/1 -> AND 1/2(input_b), AND 2/1(input_a)
  OR 2/1(output) -> NOT1/1(input_a)  "p1"
  OR 3/1(output) -> NOT2/1(input_a)  "p1"
  AND 2/1(output) -> OR 3/2(input_b)  "o1"
  NOT1/1(output) -> Memory1/1, Q/1  "t1"
  NOT2/1(output) -> Memory/1, Q not/1  "t1"
  AND 1/1(output) -> OR 2/1(input_a)  "t1"
  Memory/1 -> OR 2/2(input_b)
  Memory1/1 -> OR 3/1(input_a)

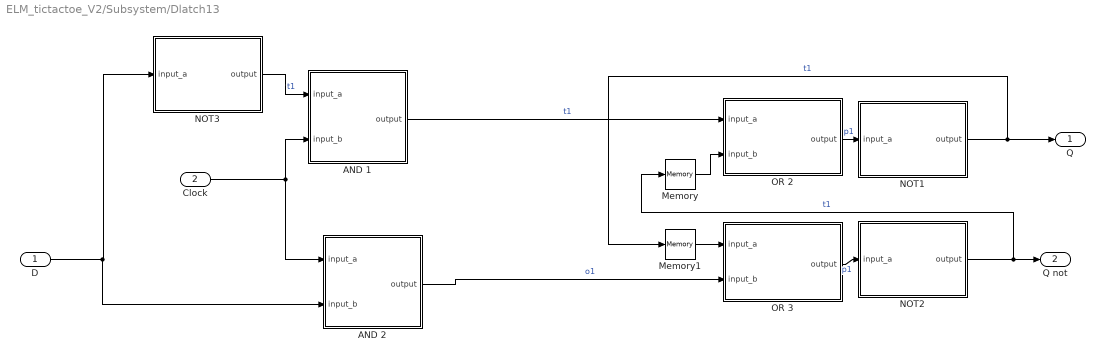
== system ELM_tictactoe_V2/Subsystem/Dlatch13 ==
  D : Inport
  Clock : Inport  Port=2
  AND 1 : MATLAB Function  TreatAsAtomicUnit=on
  AND 2 : MATLAB Function  TreatAsAtomicUnit=on
  Memory : Memory  InitialCondition=1  LinearizeAsDelay=on
  Memory1 : Memory  LinearizeAsDelay=on
  NOT1 : MATLAB Function  TreatAsAtomicUnit=on
  NOT2 : MATLAB Function  TreatAsAtomicUnit=on
  NOT3 : MATLAB Function  TreatAsAtomicUnit=on
  OR 2 : MATLAB Function  TreatAsAtomicUnit=on
  OR 3 : MATLAB Function  TreatAsAtomicUnit=on
  Q : Outport
  Q not : Outport  Port=2
  wires:
  D/1 -> NOT3/1(input_a), AND 2/2(input_b)
  NOT3/1(output) -> AND 1/1(input_a)  "t1"
  Clock/1 -> AND 1/2(input_b), AND 2/1(input_a)
  OR 2/1(output) -> NOT1/1(input_a)  "p1"
  OR 3/1(output) -> NOT2/1(input_a)  "p1"
  AND 2/1(output) -> OR 3/2(input_b)  "o1"
  NOT1/1(output) -> Memory1/1, Q/1  "t1"
  NOT2/1(output) -> Memory/1, Q not/1  "t1"
  AND 1/1(output) -> OR 2/1(input_a)  "t1"
  Memory/1 -> OR 2/2(input_b)
  Memory1/1 -> OR 3/1(input_a)

== system ELM_tictactoe_V2/Subsystem/Dlatch14 ==
  D : Inport
  Clock : Inport  Port=2
  AND 1 : MATLAB Function  TreatAsAtomicUnit=on
  AND 2 : MATLAB Function  TreatAsAtomicUnit=on
  Memory : Memory  InitialCondition=1  LinearizeAsDelay=on
  Memory1 : Memory  LinearizeAsDelay=on
  NOT1 : MATLAB Function  TreatAsAtomicUnit=on
  NOT2 : MATLAB Function  TreatAsAtomicUnit=on
  NOT3 : MATLAB Function  TreatAsAtomicUnit=on
  OR 2 : MATLAB Function  TreatAsAtomicUnit=on
  OR 3 : MATLAB Function  TreatAsAtomicUnit=on
  Q : Outport
  Q not : Outport  Port=2
  wires:
  D/1 -> NOT3/1(input_a), AND 2/2(input_b)
  NOT3/1(output) -> AND 1/1(input_a)  "t1"
  Clock/1 -> AND 1/2(input_b), AND 2/1(input_a)
  OR 2/1(output) -> NOT1/1(input_a)  "p1"
  OR 3/1(output) -> NOT2/1(input_a)  "p1"
  AND 2/1(output) -> OR 3/2(input_b)  "o1"
  NOT1/1(output) -> Memory1/1, Q/1  "t1"
  NOT2/1(output) -> Memory/1, Q not/1  "t1"
  AND 1/1(output) -> OR 2/1(input_a)  "t1"
  Memory/1 -> OR 2/2(input_b)
  Memory1/1 -> OR 3/1(input_a)

== system ELM_tictactoe_V2/Subsystem/Dlatch15 ==
  D : Inport
  Clock : Inport  Port=2
  AND 1 : MATLAB Function  TreatAsAtomicUnit=on
  AND 2 : MATLAB Function  TreatAsAtomicUnit=on
  Memory : Memory  InitialCondition=1  LinearizeAsDelay=on
  Memory1 : Memory  LinearizeAsDelay=on
  NOT1 : MATLAB Function  TreatAsAtomicUnit=on
  NOT2 : MATLAB Function  TreatAsAtomicUnit=on
  NOT3 : MATLAB Function  TreatAsAtomicUnit=on
  OR 2 : MATLAB Function  TreatAsAtomicUnit=on
  OR 3 : MATLAB Function  TreatAsAtomicUnit=on
  Q : Outport
  Q not : Outport  Port=2
  wires:
  D/1 -> NOT3/1(input_a), AND 2/2(input_b)
  NOT3/1(output) -> AND 1/1(input_a)  "t1"
  Clock/1 -> AND 1/2(input_b), AND 2/1(input_a)
  OR 2/1(output) -> NOT1/1(input_a)  "p1"
  OR 3/1(output) -> NOT2/1(input_a)  "p1"
  AND 2/1(output) -> OR 3/2(input_b)  "o1"
  NOT1/1(output) -> Memory1/1, Q/1  "t1"
  NOT2/1(output) -> Memory/1, Q not/1  "t1"
  AND 1/1(output) -> OR 2/1(input_a)  "t1"
  Memory/1 -> OR 2/2(input_b)
  Memory1/1 -> OR 3/1(input_a)

== system ELM_tictactoe_V2/Subsystem/Dlatch16 ==
  D : Inport
  Clock : Inport  Port=2
  AND 1 : MATLAB Function  TreatAsAtomicUnit=on
  AND 2 : MATLAB Function  TreatAsAtomicUnit=on
  Memory : Memory  InitialCondition=1  LinearizeAsDelay=on
  Memory1 : Memory  LinearizeAsDelay=on
  NOT1 : MATLAB Function  TreatAsAtomicUnit=on
  NOT2 : MATLAB Function  TreatAsAtomicUnit=on
  NOT3 : MATLAB Function  TreatAsAtomicUnit=on
  OR 2 : MATLAB Function  TreatAsAtomicUnit=on
  OR 3 : MATLAB Function  TreatAsAtomicUnit=on
  Q : Outport
  Q not : Outport  Port=2
  wires:
  D/1 -> NOT3/1(input_a), AND 2/2(input_b)
  NOT3/1(output) -> AND 1/1(input_a)  "t1"
  Clock/1 -> AND 1/2(input_b), AND 2/1(input_a)
  OR 2/1(output) -> NOT1/1(input_a)  "p1"
  OR 3/1(output) -> NOT2/1(input_a)  "p1"
  AND 2/1(output) -> OR 3/2(input_b)  "o1"
  NOT1/1(output) -> Memory1/1, Q/1  "t1"
  NOT2/1(output) -> Memory/1, Q not/1  "t1"
  AND 1/1(output) -> OR 2/1(input_a)  "t1"
  Memory/1 -> OR 2/2(input_b)
  Memory1/1 -> OR 3/1(input_a)

== system ELM_tictactoe_V2/Subsystem/Dlatch17 ==
  D : Inport
  Clock : Inport  Port=2
  AND 1 : MATLAB Function  TreatAsAtomicUnit=on
  AND 2 : MATLAB Function  TreatAsAtomicUnit=on
  Memory : Memory  InitialCondition=1  LinearizeAsDelay=on
  Memory1 : Memory  LinearizeAsDelay=on
  NOT1 : MATLAB Function  TreatAsAtomicUnit=on
  NOT2 : MATLAB Function  TreatAsAtomicUnit=on
  NOT3 : MATLAB Function  TreatAsAtomicUnit=on
  OR 2 : MATLAB Function  TreatAsAtomicUnit=on
  OR 3 : MATLAB Function  TreatAsAtomicUnit=on
  Q : Outport
  Q not : Outport  Port=2
  wires:
  D/1 -> NOT3/1(input_a), AND 2/2(input_b)
  NOT3/1(output) -> AND 1/1(input_a)  "t1"
  Clock/1 -> AND 1/2(input_b), AND 2/1(input_a)
  OR 2/1(output) -> NOT1/1(input_a)  "p1"
  OR 3/1(output) -> NOT2/1(input_a)  "p1"
  AND 2/1(output) -> OR 3/2(input_b)  "o1"
  NOT1/1(output) -> Memory1/1, Q/1  "t1"
  NOT2/1(output) -> Memory/1, Q not/1  "t1"
  AND 1/1(output) -> OR 2/1(input_a)  "t1"
  Memory/1 -> OR 2/2(input_b)
  Memory1/1 -> OR 3/1(input_a)

== system ELM_tictactoe_V2/Subsystem/Dlatch2 ==
  D : Inport
  Clock : Inport  Port=2
  AND 1 : MATLAB Function  TreatAsAtomicUnit=on
  AND 2 : MATLAB Function  TreatAsAtomicUnit=on
  Memory : Memory  InitialCondition=1  LinearizeAsDelay=on
  Memory1 : Memory  LinearizeAsDelay=on
  NOT1 : MATLAB Function  TreatAsAtomicUnit=on
  NOT2 : MATLAB Function  TreatAsAtomicUnit=on
  NOT3 : MATLAB Function  TreatAsAtomicUnit=on
  OR 2 : MATLAB Function  TreatAsAtomicUnit=on
  OR 3 : MATLAB Function  TreatAsAtomicUnit=on
  Q : Outport
  Q not : Outport  Port=2
  wires:
  D/1 -> NOT3/1(input_a), AND 2/2(input_b)
  NOT3/1(output) -> AND 1/1(input_a)  "t1"
  Clock/1 -> AND 1/2(input_b), AND 2/1(input_a)
  OR 2/1(output) -> NOT1/1(input_a)  "p1"
  OR 3/1(output) -> NOT2/1(input_a)  "p1"
  AND 2/1(output) -> OR 3/2(input_b)  "o1"
  NOT1/1(output) -> Memory1/1, Q/1  "t1"
  NOT2/1(output) -> Memory/1, Q not/1  "t1"
  AND 1/1(output) -> OR 2/1(input_a)  "t1"
  Memory/1 -> OR 2/2(input_b)
  Memory1/1 -> OR 3/1(input_a)

== system ELM_tictactoe_V2/Subsystem/Dlatch3 ==
  D : Inport
  Clock : Inport  Port=2
  AND 1 : MATLAB Function  TreatAsAtomicUnit=on
  AND 2 : MATLAB Function  TreatAsAtomicUnit=on
  Memory : Memory  InitialCondition=1  LinearizeAsDelay=on
  Memory1 : Memory  LinearizeAsDelay=on
  NOT1 : MATLAB Function  TreatAsAtomicUnit=on
  NOT2 : MATLAB Function  TreatAsAtomicUnit=on
  NOT3 : MATLAB Function  TreatAsAtomicUnit=on
  OR 2 : MATLAB Function  TreatAsAtomicUnit=on
  OR 3 : MATLAB Function  TreatAsAtomicUnit=on
  Q : Outport
  Q not : Outport  Port=2
  wires:
  D/1 -> NOT3/1(input_a), AND 2/2(input_b)
  NOT3/1(output) -> AND 1/1(input_a)  "t1"
  Clock/1 -> AND 1/2(input_b), AND 2/1(input_a)
  OR 2/1(output) -> NOT1/1(input_a)  "p1"
  OR 3/1(output) -> NOT2/1(input_a)  "p1"
  AND 2/1(output) -> OR 3/2(input_b)  "o1"
  NOT1/1(output) -> Memory1/1, Q/1  "t1"
  NOT2/1(output) -> Memory/1, Q not/1  "t1"
  AND 1/1(output) -> OR 2/1(input_a)  "t1"
  Memory/1 -> OR 2/2(input_b)
  Memory1/1 -> OR 3/1(input_a)

== system ELM_tictactoe_V2/Subsystem/Dlatch4 ==
  D : Inport
  Clock : Inport  Port=2
  AND 1 : MATLAB Function  TreatAsAtomicUnit=on
  AND 2 : MATLAB Function  TreatAsAtomicUnit=on
  Memory : Memory  InitialCondition=1  LinearizeAsDelay=on
  Memory1 : Memory  LinearizeAsDelay=on
  NOT1 : MATLAB Function  TreatAsAtomicUnit=on
  NOT2 : MATLAB Function  TreatAsAtomicUnit=on
  NOT3 : MATLAB Function  TreatAsAtomicUnit=on
  OR 2 : MATLAB Function  TreatAsAtomicUnit=on
  OR 3 : MATLAB Function  TreatAsAtomicUnit=on
  Q : Outport
  Q not : Outport  Port=2
  wires:
  D/1 -> NOT3/1(input_a), AND 2/2(input_b)
  NOT3/1(output) -> AND 1/1(input_a)  "t1"
  Clock/1 -> AND 1/2(input_b), AND 2/1(input_a)
  OR 2/1(output) -> NOT1/1(input_a)  "p1"
  OR 3/1(output) -> NOT2/1(input_a)  "p1"
  AND 2/1(output) -> OR 3/2(input_b)  "o1"
  NOT1/1(output) -> Memory1/1, Q/1  "t1"
  NOT2/1(output) -> Memory/1, Q not/1  "t1"
  AND 1/1(output) -> OR 2/1(input_a)  "t1"
  Memory/1 -> OR 2/2(input_b)
  Memory1/1 -> OR 3/1(input_a)

== system ELM_tictactoe_V2/Subsystem/Dlatch5 ==
  D : Inport
  Clock : Inport  Port=2
  AND 1 : MATLAB Function  TreatAsAtomicUnit=on
  AND 2 : MATLAB Function  TreatAsAtomicUnit=on
  Memory : Memory  InitialCondition=1  LinearizeAsDelay=on
  Memory1 : Memory  LinearizeAsDelay=on
  NOT1 : MATLAB Function  TreatAsAtomicUnit=on
  NOT2 : MATLAB Function  TreatAsAtomicUnit=on
  NOT3 : MATLAB Function  TreatAsAtomicUnit=on
  OR 2 : MATLAB Function  TreatAsAtomicUnit=on
  OR 3 : MATLAB Function  TreatAsAtomicUnit=on
  Q : Outport
  Q not : Outport  Port=2
  wires:
  D/1 -> NOT3/1(input_a), AND 2/2(input_b)
  NOT3/1(output) -> AND 1/1(input_a)  "t1"
  Clock/1 -> AND 1/2(input_b), AND 2/1(input_a)
  OR 2/1(output) -> NOT1/1(input_a)  "p1"
  OR 3/1(output) -> NOT2/1(input_a)  "p1"
  AND 2/1(output) -> OR 3/2(input_b)  "o1"
  NOT1/1(output) -> Memory1/1, Q/1  "t1"
  NOT2/1(output) -> Memory/1, Q not/1  "t1"
  AND 1/1(output) -> OR 2/1(input_a)  "t1"
  Memory/1 -> OR 2/2(input_b)
  Memory1/1 -> OR 3/1(input_a)

== system ELM_tictactoe_V2/Subsystem/Dlatch6 ==
  D : Inport
  Clock : Inport  Port=2
  AND 1 : MATLAB Function  TreatAsAtomicUnit=on
  AND 2 : MATLAB Function  TreatAsAtomicUnit=on
  Memory : Memory  InitialCondition=1  LinearizeAsDelay=on
  Memory1 : Memory  LinearizeAsDelay=on
  NOT1 : MATLAB Function  TreatAsAtomicUnit=on
  NOT2 : MATLAB Function  TreatAsAtomicUnit=on
  NOT3 : MATLAB Function  TreatAsAtomicUnit=on
  OR 2 : MATLAB Function  TreatAsAtomicUnit=on
  OR 3 : MATLAB Function  TreatAsAtomicUnit=on
  Q : Outport
  Q not : Outport  Port=2
  wires:
  D/1 -> NOT3/1(input_a), AND 2/2(input_b)
  NOT3/1(output) -> AND 1/1(input_a)  "t1"
  Clock/1 -> AND 1/2(input_b), AND 2/1(input_a)
  OR 2/1(output) -> NOT1/1(input_a)  "p1"
  OR 3/1(output) -> NOT2/1(input_a)  "p1"
  AND 2/1(output) -> OR 3/2(input_b)  "o1"
  NOT1/1(output) -> Memory1/1, Q/1  "t1"
  NOT2/1(output) -> Memory/1, Q not/1  "t1"
  AND 1/1(output) -> OR 2/1(input_a)  "t1"
  Memory/1 -> OR 2/2(input_b)
  Memory1/1 -> OR 3/1(input_a)

== system ELM_tictactoe_V2/Subsystem/Dlatch7 ==
  D : Inport
  Clock : Inport  Port=2
  AND 1 : MATLAB Function  TreatAsAtomicUnit=on
  AND 2 : MATLAB Function  TreatAsAtomicUnit=on
  Memory : Memory  InitialCondition=1  LinearizeAsDelay=on
  Memory1 : Memory  LinearizeAsDelay=on
  NOT1 : MATLAB Function  TreatAsAtomicUnit=on
  NOT2 : MATLAB Function  TreatAsAtomicUnit=on
  NOT3 : MATLAB Function  TreatAsAtomicUnit=on
  OR 2 : MATLAB Function  TreatAsAtomicUnit=on
  OR 3 : MATLAB Function  TreatAsAtomicUnit=on
  Q : Outport
  Q not : Outport  Port=2
  wires:
  D/1 -> NOT3/1(input_a), AND 2/2(input_b)
  NOT3/1(output) -> AND 1/1(input_a)  "t1"
  Clock/1 -> AND 1/2(input_b), AND 2/1(input_a)
  OR 2/1(output) -> NOT1/1(input_a)  "p1"
  OR 3/1(output) -> NOT2/1(input_a)  "p1"
  AND 2/1(output) -> OR 3/2(input_b)  "o1"
  NOT1/1(output) -> Memory1/1, Q/1  "t1"
  NOT2/1(output) -> Memory/1, Q not/1  "t1"
  AND 1/1(output) -> OR 2/1(input_a)  "t1"
  Memory/1 -> OR 2/2(input_b)
  Memory1/1 -> OR 3/1(input_a)

== system ELM_tictactoe_V2/Subsystem/Dlatch8 ==
  D : Inport
  Clock : Inport  Port=2
  AND 1 : MATLAB Function  TreatAsAtomicUnit=on
  AND 2 : MATLAB Function  TreatAsAtomicUnit=on
  Memory : Memory  InitialCondition=1  LinearizeAsDelay=on
  Memory1 : Memory  LinearizeAsDelay=on
  NOT1 : MATLAB Function  TreatAsAtomicUnit=on
  NOT2 : MATLAB Function  TreatAsAtomicUnit=on
  NOT3 : MATLAB Function  TreatAsAtomicUnit=on
  OR 2 : MATLAB Function  TreatAsAtomicUnit=on
  OR 3 : MATLAB Function  TreatAsAtomicUnit=on
  Q : Outport
  Q not : Outport  Port=2
  wires:
  D/1 -> NOT3/1(input_a), AND 2/2(input_b)
  NOT3/1(output) -> AND 1/1(input_a)  "t1"
  Clock/1 -> AND 1/2(input_b), AND 2/1(input_a)
  OR 2/1(output) -> NOT1/1(input_a)  "p1"
  OR 3/1(output) -> NOT2/1(input_a)  "p1"
  AND 2/1(output) -> OR 3/2(input_b)  "o1"
  NOT1/1(output) -> Memory1/1, Q/1  "t1"
  NOT2/1(output) -> Memory/1, Q not/1  "t1"
  AND 1/1(output) -> OR 2/1(input_a)  "t1"
  Memory/1 -> OR 2/2(input_b)
  Memory1/1 -> OR 3/1(input_a)

== system ELM_tictactoe_V2/Subsystem/Dlatch9 ==
  D : Inport
  Clock : Inport  Port=2
  AND 1 : MATLAB Function  TreatAsAtomicUnit=on
  AND 2 : MATLAB Function  TreatAsAtomicUnit=on
  Memory : Memory  InitialCondition=1  LinearizeAsDelay=on
  Memory1 : Memory  LinearizeAsDelay=on
  NOT1 : MATLAB Function  TreatAsAtomicUnit=on
  NOT2 : MATLAB Function  TreatAsAtomicUnit=on
  NOT3 : MATLAB Function  TreatAsAtomicUnit=on
  OR 2 : MATLAB Function  TreatAsAtomicUnit=on
  OR 3 : MATLAB Function  TreatAsAtomicUnit=on
  Q : Outport
  Q not : Outport  Port=2
  wires:
  D/1 -> NOT3/1(input_a), AND 2/2(input_b)
  NOT3/1(output) -> AND 1/1(input_a)  "t1"
  Clock/1 -> AND 1/2(input_b), AND 2/1(input_a)
  OR 2/1(output) -> NOT1/1(input_a)  "p1"
  OR 3/1(output) -> NOT2/1(input_a)  "p1"
  AND 2/1(output) -> OR 3/2(input_b)  "o1"
  NOT1/1(output) -> Memory1/1, Q/1  "t1"
  NOT2/1(output) -> Memory/1, Q not/1  "t1"
  AND 1/1(output) -> OR 2/1(input_a)  "t1"
  Memory/1 -> OR 2/2(input_b)
  Memory1/1 -> OR 3/1(input_a)

== system ELM_tictactoe_V2/Subsystem/Player Switcher a ==
  Key : Inport
  Switcher : Inport  Port=2
  AND 1 : MATLAB Function  TreatAsAtomicUnit=on
  Demultiplexer : Subsystem
      settings: PortSchema="{\"entries\":[{\"content\":{\"sides\":[{\"content\":{\"connectorIds\":[\"In1\"]},\"type\":\"ConnectorPlacement.EquallySpacedRectSide\",\"uuid\":\"6ccd7be5-9453-443a-8992-4f3046a94d81\"},{\"content\":{\"connectorIds\":[\"Out1\",\"Out2\"],\"side\":\"RIGHT\"},\"type\":\"ConnectorPlacement.EquallySpacedRectSide\",\"uuid\":\"9e3b2918-337b-479e-a737-e198b459be29\"},{\"content\":{\"connectorIds\":[],\"side\":\"TOP\"},\"type\":\"ConnectorPlacement.EquallySpacedRectSide\",\"uuid\":\"03b37edf-716a-49b3-8681-b476b437a461\"},{\"content\":{\"connectorIds\":[\"In2\"],\"side\":\"BOTTOM\"},\"type\":\"ConnectorPlacement.EquallySpacedRectSide\",\"uuid\":\"022ab476-2e55-4fe4-b85e-58af71f15e71\"}]},\"type\":\"ConnectorPlacement.EquallySpacedConnector\",\"uuid\":\"5541166b-b010-45a8-a1ab-2639d21d22e7\"}],\"packageUris\":[\"http://schema.mathworks.com/mf0/Connector/R2020b\"],\"version\":\"1.0\"}"
  Dlatch : Subsystem
  NOT : MATLAB Function  TreatAsAtomicUnit=on
  Unit Delay : UnitDelay  SampleTime=-1  HasFrameUpgradeWarning=on
  Unit Delay1 : UnitDelay  SampleTime=-1  HasFrameUpgradeWarning=on
  Unit Delay2 : UnitDelay  SampleTime=-1  HasFrameUpgradeWarning=on
  XOR5 : MATLAB Function  TreatAsAtomicUnit=on
  A : Outport
  B : Outport  Port=2
  wires:
  Key/1 -> Demultiplexer/1(Input), AND 1/1(input_a)
  Dlatch/1(Q) -> Demultiplexer/2(c)
  Demultiplexer/1(out0) -> XOR5/1(input_a), A/1
  Demultiplexer/2(out1) -> B/1, XOR5/2(input_b)
  Switcher/1 -> Dlatch/2(D)
  AND 1/1(output) -> Dlatch/1(Clock)  "o1"
  XOR5/1(output) -> NOT/1(input_a)  "o2"
  NOT/1(output) -> Unit Delay/1  "t1"
  Unit Delay/1 -> Unit Delay1/1
  Unit Delay1/1 -> Unit Delay2/1
  Unit Delay2/1 -> AND 1/2(input_b)

== system ELM_tictactoe_V2/Subsystem/Player Switcher a1 ==
  Key : Inport
  Switcher : Inport  Port=2
  AND 1 : MATLAB Function  TreatAsAtomicUnit=on
  Demultiplexer : Subsystem
      settings: PortSchema="{\"entries\":[{\"content\":{\"sides\":[{\"content\":{\"connectorIds\":[\"In1\"]},\"type\":\"ConnectorPlacement.EquallySpacedRectSide\",\"uuid\":\"6ccd7be5-9453-443a-8992-4f3046a94d81\"},{\"content\":{\"connectorIds\":[\"Out1\",\"Out2\"],\"side\":\"RIGHT\"},\"type\":\"ConnectorPlacement.EquallySpacedRectSide\",\"uuid\":\"9e3b2918-337b-479e-a737-e198b459be29\"},{\"content\":{\"connectorIds\":[],\"side\":\"TOP\"},\"type\":\"ConnectorPlacement.EquallySpacedRectSide\",\"uuid\":\"03b37edf-716a-49b3-8681-b476b437a461\"},{\"content\":{\"connectorIds\":[\"In2\"],\"side\":\"BOTTOM\"},\"type\":\"ConnectorPlacement.EquallySpacedRectSide\",\"uuid\":\"022ab476-2e55-4fe4-b85e-58af71f15e71\"}]},\"type\":\"ConnectorPlacement.EquallySpacedConnector\",\"uuid\":\"5541166b-b010-45a8-a1ab-2639d21d22e7\"}],\"packageUris\":[\"http://schema.mathworks.com/mf0/Connector/R2020b\"],\"version\":\"1.0\"}"
  Dlatch : Subsystem
  NOT : MATLAB Function  TreatAsAtomicUnit=on
  Unit Delay : UnitDelay  SampleTime=-1  HasFrameUpgradeWarning=on
  Unit Delay1 : UnitDelay  SampleTime=-1  HasFrameUpgradeWarning=on
  Unit Delay2 : UnitDelay  SampleTime=-1  HasFrameUpgradeWarning=on
  XOR5 : MATLAB Function  TreatAsAtomicUnit=on
  A : Outport
  B : Outport  Port=2
  wires:
  Key/1 -> Demultiplexer/1(Input), AND 1/1(input_a)
  Dlatch/1(Q) -> Demultiplexer/2(c)
  Demultiplexer/1(out0) -> XOR5/1(input_a), A/1
  Demultiplexer/2(out1) -> B/1, XOR5/2(input_b)
  Switcher/1 -> Dlatch/2(D)
  AND 1/1(output) -> Dlatch/1(Clock)  "o1"
  XOR5/1(output) -> NOT/1(input_a)  "o2"
  NOT/1(output) -> Unit Delay/1  "t1"
  Unit Delay/1 -> Unit Delay1/1
  Unit Delay1/1 -> Unit Delay2/1
  Unit Delay2/1 -> AND 1/2(input_b)

== system ELM_tictactoe_V2/Subsystem/Player Switcher a2 ==
  Key : Inport
  Switcher : Inport  Port=2
  AND 1 : MATLAB Function  TreatAsAtomicUnit=on
  Demultiplexer : Subsystem
      settings: PortSchema="{\"entries\":[{\"content\":{\"sides\":[{\"content\":{\"connectorIds\":[\"In1\"]},\"type\":\"ConnectorPlacement.EquallySpacedRectSide\",\"uuid\":\"6ccd7be5-9453-443a-8992-4f3046a94d81\"},{\"content\":{\"connectorIds\":[\"Out1\",\"Out2\"],\"side\":\"RIGHT\"},\"type\":\"ConnectorPlacement.EquallySpacedRectSide\",\"uuid\":\"9e3b2918-337b-479e-a737-e198b459be29\"},{\"content\":{\"connectorIds\":[],\"side\":\"TOP\"},\"type\":\"ConnectorPlacement.EquallySpacedRectSide\",\"uuid\":\"03b37edf-716a-49b3-8681-b476b437a461\"},{\"content\":{\"connectorIds\":[\"In2\"],\"side\":\"BOTTOM\"},\"type\":\"ConnectorPlacement.EquallySpacedRectSide\",\"uuid\":\"022ab476-2e55-4fe4-b85e-58af71f15e71\"}]},\"type\":\"ConnectorPlacement.EquallySpacedConnector\",\"uuid\":\"5541166b-b010-45a8-a1ab-2639d21d22e7\"}],\"packageUris\":[\"http://schema.mathworks.com/mf0/Connector/R2020b\"],\"version\":\"1.0\"}"
  Dlatch : Subsystem
  NOT : MATLAB Function  TreatAsAtomicUnit=on
  Unit Delay : UnitDelay  SampleTime=-1  HasFrameUpgradeWarning=on
  Unit Delay1 : UnitDelay  SampleTime=-1  HasFrameUpgradeWarning=on
  Unit Delay2 : UnitDelay  SampleTime=-1  HasFrameUpgradeWarning=on
  XOR5 : MATLAB Function  TreatAsAtomicUnit=on
  A : Outport
  B : Outport  Port=2
  wires:
  Key/1 -> Demultiplexer/1(Input), AND 1/1(input_a)
  Dlatch/1(Q) -> Demultiplexer/2(c)
  Demultiplexer/1(out0) -> XOR5/1(input_a), A/1
  Demultiplexer/2(out1) -> B/1, XOR5/2(input_b)
  Switcher/1 -> Dlatch/2(D)
  AND 1/1(output) -> Dlatch/1(Clock)  "o1"
  XOR5/1(output) -> NOT/1(input_a)  "o2"
  NOT/1(output) -> Unit Delay/1  "t1"
  Unit Delay/1 -> Unit Delay1/1
  Unit Delay1/1 -> Unit Delay2/1
  Unit Delay2/1 -> AND 1/2(input_b)

== system ELM_tictactoe_V2/Subsystem/Player Switcher a3 ==
  Key : Inport
  Switcher : Inport  Port=2
  AND 1 : MATLAB Function  TreatAsAtomicUnit=on
  Demultiplexer : Subsystem
      settings: PortSchema="{\"entries\":[{\"content\":{\"sides\":[{\"content\":{\"connectorIds\":[\"In1\"]},\"type\":\"ConnectorPlacement.EquallySpacedRectSide\",\"uuid\":\"6ccd7be5-9453-443a-8992-4f3046a94d81\"},{\"content\":{\"connectorIds\":[\"Out1\",\"Out2\"],\"side\":\"RIGHT\"},\"type\":\"ConnectorPlacement.EquallySpacedRectSide\",\"uuid\":\"9e3b2918-337b-479e-a737-e198b459be29\"},{\"content\":{\"connectorIds\":[],\"side\":\"TOP\"},\"type\":\"ConnectorPlacement.EquallySpacedRectSide\",\"uuid\":\"03b37edf-716a-49b3-8681-b476b437a461\"},{\"content\":{\"connectorIds\":[\"In2\"],\"side\":\"BOTTOM\"},\"type\":\"ConnectorPlacement.EquallySpacedRectSide\",\"uuid\":\"022ab476-2e55-4fe4-b85e-58af71f15e71\"}]},\"type\":\"ConnectorPlacement.EquallySpacedConnector\",\"uuid\":\"5541166b-b010-45a8-a1ab-2639d21d22e7\"}],\"packageUris\":[\"http://schema.mathworks.com/mf0/Connector/R2020b\"],\"version\":\"1.0\"}"
  Dlatch : Subsystem
  NOT : MATLAB Function  TreatAsAtomicUnit=on
  Unit Delay : UnitDelay  SampleTime=-1  HasFrameUpgradeWarning=on
  Unit Delay1 : UnitDelay  SampleTime=-1  HasFrameUpgradeWarning=on
  Unit Delay2 : UnitDelay  SampleTime=-1  HasFrameUpgradeWarning=on
  XOR5 : MATLAB Function  TreatAsAtomicUnit=on
  A : Outport
  B : Outport  Port=2
  wires:
  Key/1 -> Demultiplexer/1(Input), AND 1/1(input_a)
  Dlatch/1(Q) -> Demultiplexer/2(c)
  Demultiplexer/1(out0) -> XOR5/1(input_a), A/1
  Demultiplexer/2(out1) -> B/1, XOR5/2(input_b)
  Switcher/1 -> Dlatch/2(D)
  AND 1/1(output) -> Dlatch/1(Clock)  "o1"
  XOR5/1(output) -> NOT/1(input_a)  "o2"
  NOT/1(output) -> Unit Delay/1  "t1"
  Unit Delay/1 -> Unit Delay1/1
  Unit Delay1/1 -> Unit Delay2/1
  Unit Delay2/1 -> AND 1/2(input_b)
